simulink model "lab4"  (R2020b)
settings: Solver=VariableStepAuto  StartTime=0.0  StopTime=10.0  RelTol=1e-3
model workspace (MAT data in the model file):
  K = Simulink.Parameter
  K.Value = 0.25
  K.DataType = 'auto'
  K.Dimensions = [1 1]
settings Model: Creator=karth  LastModifiedBy=karth

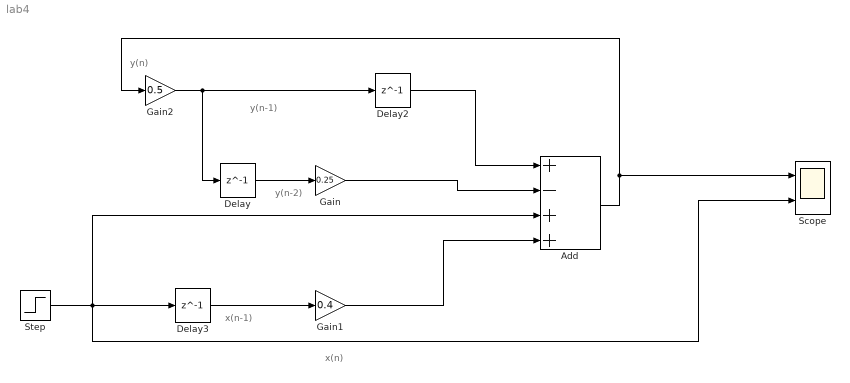
== system lab4 ==
  note: y(n)
  note: y(n-1)
  note: y(n-2)
  note: x(n-1)
  note: x(n)
  Add : Sum  Inputs=+-++
  Delay : Delay  DelayLength=1  InitialCondition=0
  Delay2 : Delay  DelayLength=1  InitialCondition=0
  Delay3 : Delay  DelayLength=1  InitialCondition=0
  Gain : Gain  Gain=0.25
  Gain1 : Gain  Gain=0.4
  Gain2 : Gain  Gain=0.5
  Scope : Scope  NumInputPorts=2
  Step : Step  SampleTime=0
  wires:
  Gain/1 -> Add/2
  Gain1/1 -> Add/4
  Delay3/1 -> Gain1/1
  Gain2/1 -> Delay/1, Delay2/1
  Delay/1 -> Gain/1
  Delay2/1 -> Add/1
  Step/1 -> Add/3, Scope/2, Delay3/1
  Add/1 -> Scope/1, Gain2/1
